simulink model "simulink_4"  (R2016a)
settings: Solver=ode5  StartTime=0.0  StopTime=10.0  FixedStep=0.01  RelTol=1e-3
settings Model: Creator=Abhay  LastModifiedBy=Abhay
settings DataIOCC: LimitDataPoints=on  SaveFormat=Array
settings DebuggingCC: SolverPrmCheckMsg=warning
settings HardwareCC: ProdBitPerPointer=32  ProdLargestAtomicFloat=None  ProdIntDivRoundTo=Undefined  ProdEndianess=Unspecified  ProdWordSize=32  ProdHWDeviceType=32-bit Generic
settings ModelReferenceCC: PropagateSignalLabelsOutOfModel=off
settings ConfigComp: CovModelRefEnable=Off  CovSFcnEnable=off

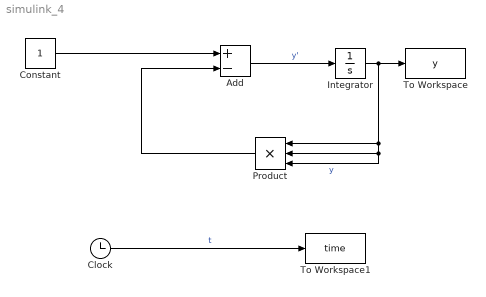
== system simulink_4 ==
  Add : Sum  Inputs=+-
  Clock : Clock
  Constant : Constant
  Integrator : Integrator  InitialCondition=-2
  Product : Product  Inputs=3
  To Workspace : ToWorkspace  VariableName=y  SampleTime=-1
  To Workspace1 : ToWorkspace  VariableName=time  SampleTime=-1
  wires:
  Constant/1 -> Add/1
  Add/1 -> Integrator/1  "y'"
  Integrator/1 -> Product/2, Product/3, Product/1, To Workspace/1  "y"
  Clock/1 -> To Workspace1/1  "t"
  Product/1 -> Add/2
